simulink model "PhyMod_CalcCor"  (R2016b)
settings: configuration reference "CodeGenConfigSet" (kept outside this file)
values from neighbouring files (symbols this model uses):
  CoEOM_facRmpVal_C = Calibration.Parameter    [init_PhyMod_CalcCor.m]
  PhyMod_facEtaCor_C = Calibration.Parameter    [init_PhyMod_CalcCor.m]
  PhyMod_facEtaCorNxt_C = Calibration.Parameter    [init_PhyMod_CalcCor.m]
  PhyMod_qCor_C = Calibration.Parameter    [init_PhyMod_CalcCor.m]
  PhyMod_qCorNxt_C = Calibration.Parameter    [init_PhyMod_CalcCor.m]
  PhyMod_stNxt_C = Calibration.Parameter    [init_PhyMod_CalcCor.m]
  PhyMod_stPrs_C = Calibration.Parameter    [init_PhyMod_CalcCor.m]
settings Model: Creator=lenovo  LastModifiedBy=lenovo
settings ConfigSetRef: SourceLocation=Base Workspace

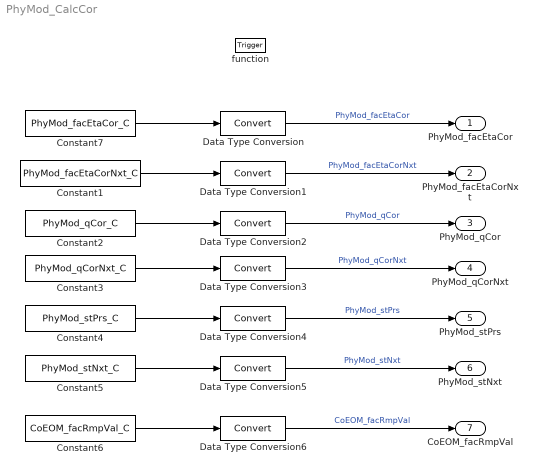
== system PhyMod_CalcCor ==
  function : TriggerPort  TriggerType=function-call  VariantControl=Variant
  Constant1 : Constant  Value=PhyMod_facEtaCorNxt_C
  Constant2 : Constant  Value=PhyMod_qCor_C
  Constant3 : Constant  Value=PhyMod_qCorNxt_C
  Constant4 : Constant  Value=PhyMod_stPrs_C
  Constant5 : Constant  Value=PhyMod_stNxt_C
  Constant6 : Constant  Value=CoEOM_facRmpVal_C
  Constant7 : Constant  Value=PhyMod_facEtaCor_C
  Data Type Conversion{,1..6} (7 alike) : DataTypeConversion
  PhyMod_facEtaCor : Outport  Description=Current efficiency correction factor  OutMin=-30  OutMax=30  OutDataTypeStr=Factor
  PhyMod_facEtaCorNxt : Outport  Description=next efficiency correction factor  Port=2  OutMin=-31  OutMax=31  OutDataTypeStr=Factor
  PhyMod_qCor : Outport  Tag=mg/hub  Description=Correction quantity  Port=3  OutMin=-319  OutMax=319  OutDataTypeStr=FuelMass_mg_hub
  PhyMod_qCorNxt : Outport  Tag=mg/hub  Description=next correction quantity  Port=4  OutMin=-319  OutMax=319  OutDataTypeStr=FuelMass_mg_hub
  PhyMod_stPrs : Outport  Description=Current operating mode for the torque structure  Port=5  OutMin=0  OutMax=255  OutDataTypeStr=State_uint8
  PhyMod_stNxt : Outport  Description=Next operating mode for the torque structure  Port=6  OutMin=0  OutMax=255  OutDataTypeStr=State_uint8
  CoEOM_facRmpVal : Outport  Description=Central ramp value for operation mode change  Port=7  OutMin=-31  OutMax=31  OutDataTypeStr=Factor
  wires:
  Data Type Conversion/1 -> PhyMod_facEtaCor/1  "PhyMod_facEtaCor"
  Data Type Conversion1/1 -> PhyMod_facEtaCorNxt/1  "PhyMod_facEtaCorNxt"
  Data Type Conversion2/1 -> PhyMod_qCor/1  "PhyMod_qCor"
  Data Type Conversion3/1 -> PhyMod_qCorNxt/1  "PhyMod_qCorNxt"
  Data Type Conversion4/1 -> PhyMod_stPrs/1  "PhyMod_stPrs"
  Data Type Conversion5/1 -> PhyMod_stNxt/1  "PhyMod_stNxt"
  Data Type Conversion6/1 -> CoEOM_facRmpVal/1  "CoEOM_facRmpVal"
  Constant1/1 -> Data Type Conversion1/1
  Constant7/1 -> Data Type Conversion/1
  Constant2/1 -> Data Type Conversion2/1
  Constant3/1 -> Data Type Conversion3/1
  Constant4/1 -> Data Type Conversion4/1
  Constant5/1 -> Data Type Conversion5/1
  Constant6/1 -> Data Type Conversion6/1
